simulink model "MPS_device_passive"  (R2018b)
settings: Solver=ode4  StartTime=0  StopTime=300  FixedStep=0.02  MaxStep=0.02  RelTol=1e-3  EnableMultiTasking=on
InitFcn:
  | %SSModel_calc
undefined symbols (not defined in the file): body, CentralPTOPreload, constraint, L, ML1Preload, ML2Preload, ML3Preload, ML4Preload, ML5Preload, ML6Preload, ML7Preload, ML8Preload, mrelative, pto, PTOrotation, SidePTO1Preload, SidePTO2Preload, SidePTO3Preload, SidePTO4Preload, simu, waves, X, Y, Z
libraries: nesl_utility x580, sm_lib x317, vrlib x72, WECSim_Lib x36
(part 2 of 27)

== system MPS_device_passive/ML4 ==
  Gimbal Fair4 : Subsystem  AncestorBlock=WECSim_Lib/Constraints/Rotational  mask(Constraints){constraint=constraint(1)}
      mask prompts: constraint "Constraint Name:"
      mask help:
      | Constraints the follower to rotational motion relative to the base, about
      | the constraint's Y-axis. Location is required and affects dynamics.
      |
      |
      | The variable name input below must be 'constraint(i)' where i=1,2,...
      | constraint(i) must be defined in the input file with the following fields:
      |
      |     .name (required)
      |             String.
      |             Constraint name. Must comply with Matlab's variable naming rules.
      |     .loc (required)
      |             3x1 vector [x y z] in meters.
      |             Constraint location. Default = [0 0 0]
      |     .orientation.z (optional)
      |             3x1 vector [x y z].
      |             Direction of the constraint's Z-coordinate. Default = [0 0 1]
      |     .orientation.y (optional)
      |             3x1 vector [x y z].
      |             Direction of the constraint's Y-coordinate. Default = [0 1 0]
      mask init: same as MPS_device_passive/Central tether/Gimbal F3
      settings: AttributesFormatString=%<constraint>
      mask Help:
      | Constraints the follower to rotational motion relative to the base, about
      | the constraint's Y-axis. Location is required and affects dynamics.
      | 
      | 
      | The variable name input below must be 'constraint(i)' where i=1,2,...
      | constraint(i) must be defined in the input file with the following fields:
      | 
      |     .name (required)
      |             String.
      |             Constraint name. Must comply with Matlab's variable naming rules.
      |     .loc (required)
      |             3x1 vector [x y z] in meters.
      |             Constraint location. Default = [0 0 0]
      |     .orientation.z (optional)
      |             3x1 vector [x y z].
      |             Direction of the constraint's Z-coordinate. Default = [0 0 1]
      |     .orientation.y (optional)
      |             3x1 vector [x y z].
      |             Direction of the constraint's Y-coordinate. Default = [0 1 0]
  ML4_preload : Constant  Value=ML4Preload
  Rigid Transform Anch4 : sm_lib/Frames and Transforms/Rigid Transform  TranslationMethod=None  TranslationStandardOffset=0  TranslationLengthUnit=m  TranslationStandardAxis=+Z  TranslationCartesianOffset=[0 0 0]  TranslationROffset=0  TranslationROffsetUnits=m  TranslationZOffset=0  TranslationZOffsetUnits=m  TranslationThetaOffset=0  TranslationThetaOffsetUnits=deg  RotationMethod=StandardAxis  RotationAngleUnits=rad  RotationStandardAxis=+Z  RotationAngle=pi-mrelative  RotationArbitraryAxis=[0 0 1]  FollAlignAxisA=+X  BaseAlignAxisA=+Y  FollAlignAxisB=+Y  BaseAlignAxisB=+Z  RotationSequenceAxes=FollowerAxes  RotationSequence=XYX  RotationSequenceAngles=[0 0 0]  RotationSequenceAnglesUnits=deg  RotationMatrix=[1 0 0; 0 1 0; 0 0 1]
  Rigid Transform F4P1 : sm_lib/Frames and Transforms/Rigid Transform  TranslationMethod=None  TranslationStandardOffset=0  TranslationLengthUnit=m  TranslationStandardAxis=+Z  TranslationCartesianOffset=[0 0 0]  TranslationROffset=0  TranslationROffsetUnits=m  TranslationZOffset=0  TranslationZOffsetUnits=m  TranslationThetaOffset=0  TranslationThetaOffsetUnits=deg  RotationMethod=StandardAxis  RotationAngleUnits=rad  RotationStandardAxis=+Z  RotationAngle=pi-mrelative  RotationArbitraryAxis=[0 0 1]  FollAlignAxisA=+X  BaseAlignAxisA=+Y  FollAlignAxisB=+Y  BaseAlignAxisB=+Z  RotationSequenceAxes=FollowerAxes  RotationSequence=XYX  RotationSequenceAngles=[0 0 0]  RotationSequenceAnglesUnits=deg  RotationMatrix=[1 0 0; 0 1 0; 0 0 1]
  Terminator3 : Terminator
  Translational PTO Actuation Force ML4 : Subsystem  AncestorBlock=WECSim_Lib/PTOs/Translational PTO Actuation Force  mask(PTO){pto=pto(9)}
      mask prompts: pto "PTO Name:"
      mask help:
      | Constraints the follower to translational motion relative to the base, in
      | the PTO's Z-direction and adds PTO stiffness and damping. Also applies a
      | user-defined force and outputs extension, velocity, and acceleration.
      |
      |
      | The variable name input below must be 'pto(i)' where i=1,2,...
      | pto(i) must be defined in the input file with the following fields:
      |
      |     .name (required)
      |             String.
      |             PTO name. Must comply with Matlab's variable naming rules.
      |     .loc (optional)
      |             3x1 vector [x y z] in meters.
      |             PTO location. Default = [0 0 0]
      |     .k (optional)
      |             Float.
      |             PTO linear spring stiffness. Default = 0
      |     .c (optional)
      |             Float.
      |             PTO linear damping coefficient. Default = 0
      |     .orientation.z (optional)
      |             3x1 vector [x y z].
      |             Direction of the PTO's Z-coordinate. Default = [0 0 1]
      |     .orientation.y (optional)
      |             3x1 vector [x y z].
      |             Direction of the PTO's Y-coordinate. Default = [0 1 0]
      mask init:
      | if exist('pto','var')
      |     h=[gcb '/output'];
      |     responseName=['pto' num2str(pto.ptoNum) '_out'];
      |     set_param(h,'VariableName',responseName);
      | end
      | 
      | pto.checkLoc('W');
      settings: AttributesFormatString=%<pto>
      mask Help:
      | Constraints the follower to translational motion relative to the base, in
      | the PTO's Z-direction and adds PTO stiffness and damping. Also applies a
      | user-defined force and outputs extension, velocity, and acceleration.
      | 
      | 
      | The variable name input below must be 'pto(i)' where i=1,2,...
      | pto(i) must be defined in the input file with the following fields:
      | 
      |     .name (required)
      |             String.
      |             PTO name. Must comply with Matlab's variable naming rules.
      |     .loc (optional)
      |             3x1 vector [x y z] in meters.
      |             PTO location. Default = [0 0 0]
      |     .k (optional)
      |             Float.
      |             PTO linear spring stiffness. Default = 0
      |     .c (optional)
      |             Float.
      |             PTO linear damping coefficient. Default = 0
      |     .orientation.z (optional)
      |             3x1 vector [x y z].
      |             Direction of the PTO's Z-coordinate. Default = [0 0 1]
      |     .orientation.y (optional)
      |             3x1 vector [x y z].
      |             Direction of the PTO's Y-coordinate. Default = [0 1 0]
  Universal Joint Anch4 : Subsystem  AncestorBlock=WECSim_Lib/Constraints/Rotational  mask(Constraints){constraint=constraint(18)}
      mask prompts: constraint "Constraint Name:"
      mask help:
      | Constraints the follower to rotational motion relative to the base, about
      | the constraint's Y-axis. Location is required and affects dynamics.
      |
      |
      | The variable name input below must be 'constraint(i)' where i=1,2,...
      | constraint(i) must be defined in the input file with the following fields:
      |
      |     .name (required)
      |             String.
      |             Constraint name. Must comply with Matlab's variable naming rules.
      |     .loc (required)
      |             3x1 vector [x y z] in meters.
      |             Constraint location. Default = [0 0 0]
      |     .orientation.z (optional)
      |             3x1 vector [x y z].
      |             Direction of the constraint's Z-coordinate. Default = [0 0 1]
      |     .orientation.y (optional)
      |             3x1 vector [x y z].
      |             Direction of the constraint's Y-coordinate. Default = [0 1 0]
      mask init: same as MPS_device_passive/Central tether/Gimbal F3
      settings: AttributesFormatString=%<constraint>
      mask Help:
      | Constraints the follower to rotational motion relative to the base, about
      | the constraint's Y-axis. Location is required and affects dynamics.
      | 
      | 
      | The variable name input below must be 'constraint(i)' where i=1,2,...
      | constraint(i) must be defined in the input file with the following fields:
      | 
      |     .name (required)
      |             String.
      |             Constraint name. Must comply with Matlab's variable naming rules.
      |     .loc (required)
      |             3x1 vector [x y z] in meters.
      |             Constraint location. Default = [0 0 0]
      |     .orientation.z (optional)
      |             3x1 vector [x y z].
      |             Direction of the constraint's Z-coordinate. Default = [0 0 1]
      |     .orientation.y (optional)
      |             3x1 vector [x y z].
      |             Direction of the constraint's Y-coordinate. Default = [0 1 0]
  VisuML1 : WECSim_Lib/Body Elements/Rigid Body  body=body(28)
      settings: AttributesFormatString=%<body>  SourceProductName=WEC-Sim
  VisuML2 : WECSim_Lib/Body Elements/Rigid Body  body=body(29)
      settings: AttributesFormatString=%<body>  SourceProductName=WEC-Sim
  VisuML4 : WECSim_Lib/Body Elements/Rigid Body  body=body(27)
      settings: AttributesFormatString=%<body>  SourceProductName=WEC-Sim
  Conn1 : PMIOPort  Side=Right
  Conn2 : PMIOPort  Port=2  Side=Left
  wires:
  ML4_preload/1 -> Translational PTO Actuation Force ML4/1(Force)
  Translational PTO Actuation Force ML4/1(Response) -> Terminator3/1
  connections:
  Gimbal Fair4/LConn1 -- Translational PTO Actuation Force ML4/RConn1 -- VisuML4/RConn1
  Rigid Transform F4P1/RConn1 -- Gimbal Fair4/RConn1
  Translational PTO Actuation Force ML4/LConn1 -- VisuML2/RConn1 -- Universal Joint Anch4/RConn1
  Universal Joint Anch4/LConn1 -- Rigid Transform Anch4/RConn1
  Rigid Transform F4P1/LConn1 -- VisuML1/RConn1 -- Conn2/RConn1
  Rigid Transform Anch4/LConn1 -- Conn1/RConn1

== system MPS_device_passive/ML5ver ==
  Gimbal Fair5 : Subsystem  AncestorBlock=WECSim_Lib/Constraints/Rotational  mask(Constraints){constraint=constraint(20)}
      mask prompts: constraint "Constraint Name:"
      mask help:
      | Constraints the follower to rotational motion relative to the base, about
      | the constraint's Y-axis. Location is required and affects dynamics.
      |
      |
      | The variable name input below must be 'constraint(i)' where i=1,2,...
      | constraint(i) must be defined in the input file with the following fields:
      |
      |     .name (required)
      |             String.
      |             Constraint name. Must comply with Matlab's variable naming rules.
      |     .loc (required)
      |             3x1 vector [x y z] in meters.
      |             Constraint location. Default = [0 0 0]
      |     .orientation.z (optional)
      |             3x1 vector [x y z].
      |             Direction of the constraint's Z-coordinate. Default = [0 0 1]
      |     .orientation.y (optional)
      |             3x1 vector [x y z].
      |             Direction of the constraint's Y-coordinate. Default = [0 1 0]
      mask init: same as MPS_device_passive/Central tether/Gimbal F3
      settings: AttributesFormatString=%<constraint>
      mask Help:
      | Constraints the follower to rotational motion relative to the base, about
      | the constraint's Y-axis. Location is required and affects dynamics.
      | 
      | 
      | The variable name input below must be 'constraint(i)' where i=1,2,...
      | constraint(i) must be defined in the input file with the following fields:
      | 
      |     .name (required)
      |             String.
      |             Constraint name. Must comply with Matlab's variable naming rules.
      |     .loc (required)
      |             3x1 vector [x y z] in meters.
      |             Constraint location. Default = [0 0 0]
      |     .orientation.z (optional)
      |             3x1 vector [x y z].
      |             Direction of the constraint's Z-coordinate. Default = [0 0 1]
      |     .orientation.y (optional)
      |             3x1 vector [x y z].
      |             Direction of the constraint's Y-coordinate. Default = [0 1 0]
  ML5_preload : Constant  Value=ML5Preload
  Rigid Transform Anch5 : sm_lib/Frames and Transforms/Rigid Transform  TranslationMethod=None  TranslationStandardOffset=0  TranslationLengthUnit=m  TranslationStandardAxis=+Z  TranslationCartesianOffset=[0 0 0]  TranslationROffset=0  TranslationROffsetUnits=m  TranslationZOffset=0  TranslationZOffsetUnits=m  TranslationThetaOffset=0  TranslationThetaOffsetUnits=deg  RotationMethod=StandardAxis  RotationAngleUnits=rad  RotationStandardAxis=+Z  RotationAngle=mrelative  RotationArbitraryAxis=[0 0 1]  FollAlignAxisA=+X  BaseAlignAxisA=+Y  FollAlignAxisB=+Y  BaseAlignAxisB=+Z  RotationSequenceAxes=FollowerAxes  RotationSequence=XYX  RotationSequenceAngles=[0 0 0]  RotationSequenceAnglesUnits=deg  RotationMatrix=[1 0 0; 0 1 0; 0 0 1]
  Rigid Transform Fair6 : sm_lib/Frames and Transforms/Rigid Transform  TranslationMethod=None  TranslationStandardOffset=0  TranslationLengthUnit=m  TranslationStandardAxis=+Z  TranslationCartesianOffset=[0 0 0]  TranslationROffset=0  TranslationROffsetUnits=m  TranslationZOffset=0  TranslationZOffsetUnits=m  TranslationThetaOffset=0  TranslationThetaOffsetUnits=deg  RotationMethod=StandardAxis  RotationAngleUnits=rad  RotationStandardAxis=+Z  RotationAngle=mrelative  RotationArbitraryAxis=[0 0 1]  FollAlignAxisA=+X  BaseAlignAxisA=+Y  FollAlignAxisB=+Y  BaseAlignAxisB=+Z  RotationSequenceAxes=FollowerAxes  RotationSequence=XYX  RotationSequenceAngles=[0 0 0]  RotationSequenceAnglesUnits=deg  RotationMatrix=[1 0 0; 0 1 0; 0 0 1]
  Terminator : Terminator
  Translational Actuation Force ML5 : Subsystem  AncestorBlock=WECSim_Lib/PTOs/Translational PTO Actuation Force  mask(PTO){pto=pto(10)}
      mask prompts: pto "PTO Name:"
      mask help:
      | Constraints the follower to translational motion relative to the base, in
      | the PTO's Z-direction and adds PTO stiffness and damping. Also applies a
      | user-defined force and outputs extension, velocity, and acceleration.
      |
      |
      | The variable name input below must be 'pto(i)' where i=1,2,...
      | pto(i) must be defined in the input file with the following fields:
      |
      |     .name (required)
      |             String.
      |             PTO name. Must comply with Matlab's variable naming rules.
      |     .loc (optional)
      |             3x1 vector [x y z] in meters.
      |             PTO location. Default = [0 0 0]
      |     .k (optional)
      |             Float.
      |             PTO linear spring stiffness. Default = 0
      |     .c (optional)
      |             Float.
      |             PTO linear damping coefficient. Default = 0
      |     .orientation.z (optional)
      |             3x1 vector [x y z].
      |             Direction of the PTO's Z-coordinate. Default = [0 0 1]
      |     .orientation.y (optional)
      |             3x1 vector [x y z].
      |             Direction of the PTO's Y-coordinate. Default = [0 1 0]
      mask init:
      | if exist('pto','var')
      |     h=[gcb '/output'];
      |     responseName=['pto' num2str(pto.ptoNum) '_out'];
      |     set_param(h,'VariableName',responseName);
      | end
      | 
      | pto.checkLoc('W');
      settings: AttributesFormatString=%<pto>
      mask Help:
      | Constraints the follower to translational motion relative to the base, in
      | the PTO's Z-direction and adds PTO stiffness and damping. Also applies a
      | user-defined force and outputs extension, velocity, and acceleration.
      | 
      | 
      | The variable name input below must be 'pto(i)' where i=1,2,...
      | pto(i) must be defined in the input file with the following fields:
      | 
      |     .name (required)
      |             String.
      |             PTO name. Must comply with Matlab's variable naming rules.
      |     .loc (optional)
      |             3x1 vector [x y z] in meters.
      |             PTO location. Default = [0 0 0]
      |     .k (optional)
      |             Float.
      |             PTO linear spring stiffness. Default = 0
      |     .c (optional)
      |             Float.
      |             PTO linear damping coefficient. Default = 0
      |     .orientation.z (optional)
      |             3x1 vector [x y z].
      |             Direction of the PTO's Z-coordinate. Default = [0 0 1]
      |     .orientation.y (optional)
      |             3x1 vector [x y z].
      |             Direction of the PTO's Y-coordinate. Default = [0 1 0]
  Universal Joint Anch5 : Subsystem  AncestorBlock=WECSim_Lib/Constraints/Rotational  mask(Constraints){constraint=constraint(19)}
      mask prompts: constraint "Constraint Name:"
      mask help:
      | Constraints the follower to rotational motion relative to the base, about
      | the constraint's Y-axis. Location is required and affects dynamics.
      |
      |
      | The variable name input below must be 'constraint(i)' where i=1,2,...
      | constraint(i) must be defined in the input file with the following fields:
      |
      |     .name (required)
      |             String.
      |             Constraint name. Must comply with Matlab's variable naming rules.
      |     .loc (required)
      |             3x1 vector [x y z] in meters.
      |             Constraint location. Default = [0 0 0]
      |     .orientation.z (optional)
      |             3x1 vector [x y z].
      |             Direction of the constraint's Z-coordinate. Default = [0 0 1]
      |     .orientation.y (optional)
      |             3x1 vector [x y z].
      |             Direction of the constraint's Y-coordinate. Default = [0 1 0]
      mask init: same as MPS_device_passive/Central tether/Gimbal F3
      settings: AttributesFormatString=%<constraint>
      mask Help:
      | Constraints the follower to rotational motion relative to the base, about
      | the constraint's Y-axis. Location is required and affects dynamics.
      | 
      | 
      | The variable name input below must be 'constraint(i)' where i=1,2,...
      | constraint(i) must be defined in the input file with the following fields:
      | 
      |     .name (required)
      |             String.
      |             Constraint name. Must comply with Matlab's variable naming rules.
      |     .loc (required)
      |             3x1 vector [x y z] in meters.
      |             Constraint location. Default = [0 0 0]
      |     .orientation.z (optional)
      |             3x1 vector [x y z].
      |             Direction of the constraint's Z-coordinate. Default = [0 0 1]
      |     .orientation.y (optional)
      |             3x1 vector [x y z].
      |             Direction of the constraint's Y-coordinate. Default = [0 1 0]
  VisuML5_1 : WECSim_Lib/Body Elements/Rigid Body  body=body(30)
      settings: AttributesFormatString=%<body>  SourceProductName=WEC-Sim
  VisuML5_2 : WECSim_Lib/Body Elements/Rigid Body  body=body(31)
      settings: AttributesFormatString=%<body>  SourceProductName=WEC-Sim
  VisuML5_3 : WECSim_Lib/Body Elements/Rigid Body  body=body(32)
      settings: AttributesFormatString=%<body>  SourceProductName=WEC-Sim
  Conn1 : PMIOPort  Side=Right
  Conn2 : PMIOPort  Port=2  Side=Left
  wires:
  Translational Actuation Force ML5/1(Response) -> Terminator/1
  ML5_preload/1 -> Translational Actuation Force ML5/1(Force)
  connections:
  VisuML5_1/RConn1 -- Translational Actuation Force ML5/RConn1 -- Gimbal Fair5/LConn1
  Translational Actuation Force ML5/LConn1 -- VisuML5_3/RConn1 -- Universal Joint Anch5/RConn1
  Universal Joint Anch5/LConn1 -- Rigid Transform Anch5/RConn1
  Rigid Transform Fair6/RConn1 -- Gimbal Fair5/RConn1
  Conn1/RConn1 -- Rigid Transform Anch5/LConn1
  Conn2/RConn1 -- VisuML5_2/RConn1 -- Rigid Transform Fair6/LConn1

== system MPS_device_passive/ML6ver ==
  Gimbal Fair6 : Subsystem  AncestorBlock=WECSim_Lib/Constraints/Rotational  mask(Constraints){constraint=constraint(22)}
      mask prompts: constraint "Constraint Name:"
      mask help:
      | Constraints the follower to rotational motion relative to the base, about
      | the constraint's Y-axis. Location is required and affects dynamics.
      |
      |
      | The variable name input below must be 'constraint(i)' where i=1,2,...
      | constraint(i) must be defined in the input file with the following fields:
      |
      |     .name (required)
      |             String.
      |             Constraint name. Must comply with Matlab's variable naming rules.
      |     .loc (required)
      |             3x1 vector [x y z] in meters.
      |             Constraint location. Default = [0 0 0]
      |     .orientation.z (optional)
      |             3x1 vector [x y z].
      |             Direction of the constraint's Z-coordinate. Default = [0 0 1]
      |     .orientation.y (optional)
      |             3x1 vector [x y z].
      |             Direction of the constraint's Y-coordinate. Default = [0 1 0]
      mask init: same as MPS_device_passive/Central tether/Gimbal F3
      settings: AttributesFormatString=%<constraint>
      mask Help:
      | Constraints the follower to rotational motion relative to the base, about
      | the constraint's Y-axis. Location is required and affects dynamics.
      | 
      | 
      | The variable name input below must be 'constraint(i)' where i=1,2,...
      | constraint(i) must be defined in the input file with the following fields:
      | 
      |     .name (required)
      |             String.
      |             Constraint name. Must comply with Matlab's variable naming rules.
      |     .loc (required)
      |             3x1 vector [x y z] in meters.
      |             Constraint location. Default = [0 0 0]
      |     .orientation.z (optional)
      |             3x1 vector [x y z].
      |             Direction of the constraint's Z-coordinate. Default = [0 0 1]
      |     .orientation.y (optional)
      |             3x1 vector [x y z].
      |             Direction of the constraint's Y-coordinate. Default = [0 1 0]
  ML6_preload : Constant  Value=ML6Preload
  Rigid Transform Anch6 : sm_lib/Frames and Transforms/Rigid Transform  TranslationMethod=None  TranslationStandardOffset=0  TranslationLengthUnit=m  TranslationStandardAxis=+Z  TranslationCartesianOffset=[0 0 0]  TranslationROffset=0  TranslationROffsetUnits=m  TranslationZOffset=0  TranslationZOffsetUnits=m  TranslationThetaOffset=0  TranslationThetaOffsetUnits=deg  RotationMethod=StandardAxis  RotationAngleUnits=rad  RotationStandardAxis=+Z  RotationAngle=-mrelative  RotationArbitraryAxis=[0 0 1]  FollAlignAxisA=+X  BaseAlignAxisA=+Y  FollAlignAxisB=+Y  BaseAlignAxisB=+Z  RotationSequenceAxes=FollowerAxes  RotationSequence=XYX  RotationSequenceAngles=[0 0 0]  RotationSequenceAnglesUnits=deg  RotationMatrix=[1 0 0; 0 1 0; 0 0 1]
  Rigid Transform Fair7 : sm_lib/Frames and Transforms/Rigid Transform  TranslationMethod=None  TranslationStandardOffset=0  TranslationLengthUnit=m  TranslationStandardAxis=+Z  TranslationCartesianOffset=[0 0 0]  TranslationROffset=0  TranslationROffsetUnits=m  TranslationZOffset=0  TranslationZOffsetUnits=m  TranslationThetaOffset=0  TranslationThetaOffsetUnits=deg  RotationMethod=StandardAxis  RotationAngleUnits=rad  RotationStandardAxis=+Z  RotationAngle=-mrelative  RotationArbitraryAxis=[0 0 1]  FollAlignAxisA=+X  BaseAlignAxisA=+Y  FollAlignAxisB=+Y  BaseAlignAxisB=+Z  RotationSequenceAxes=FollowerAxes  RotationSequence=XYX  RotationSequenceAngles=[0 0 0]  RotationSequenceAnglesUnits=deg  RotationMatrix=[1 0 0; 0 1 0; 0 0 1]
  Terminator1 : Terminator
  Translational PTO Actuation Force ML6 : Subsystem  AncestorBlock=WECSim_Lib/PTOs/Translational PTO Actuation Force  mask(PTO){pto=pto(11)}
      mask prompts: pto "PTO Name:"
      mask help:
      | Constraints the follower to translational motion relative to the base, in
      | the PTO's Z-direction and adds PTO stiffness and damping. Also applies a
      | user-defined force and outputs extension, velocity, and acceleration.
      |
      |
      | The variable name input below must be 'pto(i)' where i=1,2,...
      | pto(i) must be defined in the input file with the following fields:
      |
      |     .name (required)
      |             String.
      |             PTO name. Must comply with Matlab's variable naming rules.
      |     .loc (optional)
      |             3x1 vector [x y z] in meters.
      |             PTO location. Default = [0 0 0]
      |     .k (optional)
      |             Float.
      |             PTO linear spring stiffness. Default = 0
      |     .c (optional)
      |             Float.
      |             PTO linear damping coefficient. Default = 0
      |     .orientation.z (optional)
      |             3x1 vector [x y z].
      |             Direction of the PTO's Z-coordinate. Default = [0 0 1]
      |     .orientation.y (optional)
      |             3x1 vector [x y z].
      |             Direction of the PTO's Y-coordinate. Default = [0 1 0]
      mask init:
      | if exist('pto','var')
      |     h=[gcb '/output'];
      |     responseName=['pto' num2str(pto.ptoNum) '_out'];
      |     set_param(h,'VariableName',responseName);
      | end
      | 
      | pto.checkLoc('W');
      settings: AttributesFormatString=%<pto>
      mask Help:
      | Constraints the follower to translational motion relative to the base, in
      | the PTO's Z-direction and adds PTO stiffness and damping. Also applies a
      | user-defined force and outputs extension, velocity, and acceleration.
      | 
      | 
      | The variable name input below must be 'pto(i)' where i=1,2,...
      | pto(i) must be defined in the input file with the following fields:
      | 
      |     .name (required)
      |             String.
      |             PTO name. Must comply with Matlab's variable naming rules.
      |     .loc (optional)
      |             3x1 vector [x y z] in meters.
      |             PTO location. Default = [0 0 0]
      |     .k (optional)
      |             Float.
      |             PTO linear spring stiffness. Default = 0
      |     .c (optional)
      |             Float.
      |             PTO linear damping coefficient. Default = 0
      |     .orientation.z (optional)
      |             3x1 vector [x y z].
      |             Direction of the PTO's Z-coordinate. Default = [0 0 1]
      |     .orientation.y (optional)
      |             3x1 vector [x y z].
      |             Direction of the PTO's Y-coordinate. Default = [0 1 0]
  Universal Joint Anch6 : Subsystem  AncestorBlock=WECSim_Lib/Constraints/Rotational  mask(Constraints){constraint=constraint(21)}
      mask prompts: constraint "Constraint Name:"
      mask help:
      | Constraints the follower to rotational motion relative to the base, about
      | the constraint's Y-axis. Location is required and affects dynamics.
      |
      |
      | The variable name input below must be 'constraint(i)' where i=1,2,...
      | constraint(i) must be defined in the input file with the following fields:
      |
      |     .name (required)
      |             String.
      |             Constraint name. Must comply with Matlab's variable naming rules.
      |     .loc (required)
      |             3x1 vector [x y z] in meters.
      |             Constraint location. Default = [0 0 0]
      |     .orientation.z (optional)
      |             3x1 vector [x y z].
      |             Direction of the constraint's Z-coordinate. Default = [0 0 1]
      |     .orientation.y (optional)
      |             3x1 vector [x y z].
      |             Direction of the constraint's Y-coordinate. Default = [0 1 0]
      mask init: same as MPS_device_passive/Central tether/Gimbal F3
      settings: AttributesFormatString=%<constraint>
      mask Help:
      | Constraints the follower to rotational motion relative to the base, about
      | the constraint's Y-axis. Location is required and affects dynamics.
      | 
      | 
      | The variable name input below must be 'constraint(i)' where i=1,2,...
      | constraint(i) must be defined in the input file with the following fields:
      | 
      |     .name (required)
      |             String.
      |             Constraint name. Must comply with Matlab's variable naming rules.
      |     .loc (required)
      |             3x1 vector [x y z] in meters.
      |             Constraint location. Default = [0 0 0]
      |     .orientation.z (optional)
      |             3x1 vector [x y z].
      |             Direction of the constraint's Z-coordinate. Default = [0 0 1]
      |     .orientation.y (optional)
      |             3x1 vector [x y z].
      |             Direction of the constraint's Y-coordinate. Default = [0 1 0]
  VisuML6_1 : WECSim_Lib/Body Elements/Rigid Body  body=body(33)
      settings: AttributesFormatString=%<body>  SourceProductName=WEC-Sim
  VisuML6_2 : WECSim_Lib/Body Elements/Rigid Body  body=body(34)
      settings: AttributesFormatString=%<body>  SourceProductName=WEC-Sim
  VisuML6_3 : WECSim_Lib/Body Elements/Rigid Body  body=body(35)
      settings: AttributesFormatString=%<body>  SourceProductName=WEC-Sim
  Conn1 : PMIOPort  Side=Right
  Conn2 : PMIOPort  Port=2  Side=Left
  wires:
  ML6_preload/1 -> Translational PTO Actuation Force ML6/1(Force)
  Translational PTO Actuation Force ML6/1(Response) -> Terminator1/1
  connections:
  VisuML6_1/RConn1 -- Translational PTO Actuation Force ML6/RConn1 -- Gimbal Fair6/LConn1
  Rigid Transform Fair7/RConn1 -- Gimbal Fair6/RConn1
  Translational PTO Actuation Force ML6/LConn1 -- VisuML6_3/RConn1 -- Universal Joint Anch6/RConn1
  Universal Joint Anch6/LConn1 -- Rigid Transform Anch6/RConn1
  Conn1/RConn1 -- Rigid Transform Anch6/LConn1
  Conn2/RConn1 -- Rigid Transform Fair7/LConn1 -- VisuML6_2/RConn1

== system MPS_device_passive/ML7ver ==
  Gimbal Fair7 : Subsystem  AncestorBlock=WECSim_Lib/Constraints/Rotational  mask(Constraints){constraint=constraint(24)}
      mask prompts: constraint "Constraint Name:"
      mask help:
      | Constraints the follower to rotational motion relative to the base, about
      | the constraint's Y-axis. Location is required and affects dynamics.
      |
      |
      | The variable name input below must be 'constraint(i)' where i=1,2,...
      | constraint(i) must be defined in the input file with the following fields:
      |
      |     .name (required)
      |             String.
      |             Constraint name. Must comply with Matlab's variable naming rules.
      |     .loc (required)
      |             3x1 vector [x y z] in meters.
      |             Constraint location. Default = [0 0 0]
      |     .orientation.z (optional)
      |             3x1 vector [x y z].
      |             Direction of the constraint's Z-coordinate. Default = [0 0 1]
      |     .orientation.y (optional)
      |             3x1 vector [x y z].
      |             Direction of the constraint's Y-coordinate. Default = [0 1 0]
      mask init: same as MPS_device_passive/Central tether/Gimbal F3
      settings: AttributesFormatString=%<constraint>
      mask Help:
      | Constraints the follower to rotational motion relative to the base, about
      | the constraint's Y-axis. Location is required and affects dynamics.
      | 
      | 
      | The variable name input below must be 'constraint(i)' where i=1,2,...
      | constraint(i) must be defined in the input file with the following fields:
      | 
      |     .name (required)
      |             String.
      |             Constraint name. Must comply with Matlab's variable naming rules.
      |     .loc (required)
      |             3x1 vector [x y z] in meters.
      |             Constraint location. Default = [0 0 0]
      |     .orientation.z (optional)
      |             3x1 vector [x y z].
      |             Direction of the constraint's Z-coordinate. Default = [0 0 1]
      |     .orientation.y (optional)
      |             3x1 vector [x y z].
      |             Direction of the constraint's Y-coordinate. Default = [0 1 0]
  ML7_preload : Constant  Value=ML7Preload
  Rigid Transform Anch7 : sm_lib/Frames and Transforms/Rigid Transform  TranslationMethod=None  TranslationStandardOffset=0  TranslationLengthUnit=m  TranslationStandardAxis=+Z  TranslationCartesianOffset=[0 0 0]  TranslationROffset=0  TranslationROffsetUnits=m  TranslationZOffset=0  TranslationZOffsetUnits=m  TranslationThetaOffset=0  TranslationThetaOffsetUnits=deg  RotationMethod=StandardAxis  RotationAngleUnits=rad  RotationStandardAxis=+Z  RotationAngle=-pi+mrelative  RotationArbitraryAxis=[0 0 1]  FollAlignAxisA=+X  BaseAlignAxisA=+Y  FollAlignAxisB=+Y  BaseAlignAxisB=+Z  RotationSequenceAxes=FollowerAxes  RotationSequence=XYX  RotationSequenceAngles=[0 0 0]  RotationSequenceAnglesUnits=deg  RotationMatrix=[1 0 0; 0 1 0; 0 0 1]
  Rigid Transform Fair8 : sm_lib/Frames and Transforms/Rigid Transform  TranslationMethod=None  TranslationStandardOffset=0  TranslationLengthUnit=m  TranslationStandardAxis=+Z  TranslationCartesianOffset=[0 0 0]  TranslationROffset=0  TranslationROffsetUnits=m  TranslationZOffset=0  TranslationZOffsetUnits=m  TranslationThetaOffset=0  TranslationThetaOffsetUnits=deg  RotationMethod=StandardAxis  RotationAngleUnits=rad  RotationStandardAxis=+Z  RotationAngle=-pi+mrelative  RotationArbitraryAxis=[0 0 1]  FollAlignAxisA=+X  BaseAlignAxisA=+Y  FollAlignAxisB=+Y  BaseAlignAxisB=+Z  RotationSequenceAxes=FollowerAxes  RotationSequence=XYX  RotationSequenceAngles=[0 0 0]  RotationSequenceAnglesUnits=deg  RotationMatrix=[1 0 0; 0 1 0; 0 0 1]
  Terminator2 : Terminator
  Translational PTO Actuation Force ML7 : Subsystem  AncestorBlock=WECSim_Lib/PTOs/Translational PTO Actuation Force  mask(PTO){pto=pto(12)}
      mask prompts: pto "PTO Name:"
      mask help:
      | Constraints the follower to translational motion relative to the base, in
      | the PTO's Z-direction and adds PTO stiffness and damping. Also applies a
      | user-defined force and outputs extension, velocity, and acceleration.
      |
      |
      | The variable name input below must be 'pto(i)' where i=1,2,...
      | pto(i) must be defined in the input file with the following fields:
      |
      |     .name (required)
      |             String.
      |             PTO name. Must comply with Matlab's variable naming rules.
      |     .loc (optional)
      |             3x1 vector [x y z] in meters.
      |             PTO location. Default = [0 0 0]
      |     .k (optional)
      |             Float.
      |             PTO linear spring stiffness. Default = 0
      |     .c (optional)
      |             Float.
      |             PTO linear damping coefficient. Default = 0
      |     .orientation.z (optional)
      |             3x1 vector [x y z].
      |             Direction of the PTO's Z-coordinate. Default = [0 0 1]
      |     .orientation.y (optional)
      |             3x1 vector [x y z].
      |             Direction of the PTO's Y-coordinate. Default = [0 1 0]
      mask init:
      | if exist('pto','var')
      |     h=[gcb '/output'];
      |     responseName=['pto' num2str(pto.ptoNum) '_out'];
      |     set_param(h,'VariableName',responseName);
      | end
      | 
      | pto.checkLoc('W');
      settings: AttributesFormatString=%<pto>
      mask Help:
      | Constraints the follower to translational motion relative to the base, in
      | the PTO's Z-direction and adds PTO stiffness and damping. Also applies a
      | user-defined force and outputs extension, velocity, and acceleration.
      | 
      | 
      | The variable name input below must be 'pto(i)' where i=1,2,...
      | pto(i) must be defined in the input file with the following fields:
      | 
      |     .name (required)
      |             String.
      |             PTO name. Must comply with Matlab's variable naming rules.
      |     .loc (optional)
      |             3x1 vector [x y z] in meters.
      |             PTO location. Default = [0 0 0]
      |     .k (optional)
      |             Float.
      |             PTO linear spring stiffness. Default = 0
      |     .c (optional)
      |             Float.
      |             PTO linear damping coefficient. Default = 0
      |     .orientation.z (optional)
      |             3x1 vector [x y z].
      |             Direction of the PTO's Z-coordinate. Default = [0 0 1]
      |     .orientation.y (optional)
      |             3x1 vector [x y z].
      |             Direction of the PTO's Y-coordinate. Default = [0 1 0]
  Universal Joint Anch7 : Subsystem  AncestorBlock=WECSim_Lib/Constraints/Rotational  mask(Constraints){constraint=constraint(23)}
      mask prompts: constraint "Constraint Name:"
      mask help:
      | Constraints the follower to rotational motion relative to the base, about
      | the constraint's Y-axis. Location is required and affects dynamics.
      |
      |
      | The variable name input below must be 'constraint(i)' where i=1,2,...
      | constraint(i) must be defined in the input file with the following fields:
      |
      |     .name (required)
      |             String.
      |             Constraint name. Must comply with Matlab's variable naming rules.
      |     .loc (required)
      |             3x1 vector [x y z] in meters.
      |             Constraint location. Default = [0 0 0]
      |     .orientation.z (optional)
      |             3x1 vector [x y z].
      |             Direction of the constraint's Z-coordinate. Default = [0 0 1]
      |     .orientation.y (optional)
      |             3x1 vector [x y z].
      |             Direction of the constraint's Y-coordinate. Default = [0 1 0]
      mask init: same as MPS_device_passive/Central tether/Gimbal F3
      settings: AttributesFormatString=%<constraint>
      mask Help:
      | Constraints the follower to rotational motion relative to the base, about
      | the constraint's Y-axis. Location is required and affects dynamics.
      | 
      | 
      | The variable name input below must be 'constraint(i)' where i=1,2,...
      | constraint(i) must be defined in the input file with the following fields:
      | 
      |     .name (required)
      |             String.
      |             Constraint name. Must comply with Matlab's variable naming rules.
      |     .loc (required)
      |             3x1 vector [x y z] in meters.
      |             Constraint location. Default = [0 0 0]
      |     .orientation.z (optional)
      |             3x1 vector [x y z].
      |             Direction of the constraint's Z-coordinate. Default = [0 0 1]
      |     .orientation.y (optional)
      |             3x1 vector [x y z].
      |             Direction of the constraint's Y-coordinate. Default = [0 1 0]
  VisuML7_1 : WECSim_Lib/Body Elements/Rigid Body  body=body(36)
      settings: AttributesFormatString=%<body>  SourceProductName=WEC-Sim
  VisuML7_2 : WECSim_Lib/Body Elements/Rigid Body  body=body(37)
      settings: AttributesFormatString=%<body>  SourceProductName=WEC-Sim
  VisuML7_3 : WECSim_Lib/Body Elements/Rigid Body  body=body(38)
      settings: AttributesFormatString=%<body>  SourceProductName=WEC-Sim
  Conn1 : PMIOPort  Side=Right
  Conn2 : PMIOPort  Port=2  Side=Left
  wires:
  Translational PTO Actuation Force ML7/1(Response) -> Terminator2/1
  ML7_preload/1 -> Translational PTO Actuation Force ML7/1(Force1)
  connections:
  Gimbal Fair7/LConn1 -- Translational PTO Actuation Force ML7/RConn1 -- VisuML7_1/RConn1
  Rigid Transform Fair8/RConn1 -- Gimbal Fair7/RConn1
  Translational PTO Actuation Force ML7/LConn1 -- VisuML7_3/RConn1 -- Universal Joint Anch7/RConn1
  Universal Joint Anch7/LConn1 -- Rigid Transform Anch7/RConn1
  Conn1/RConn1 -- Rigid Transform Anch7/LConn1
  Conn2/RConn1 -- VisuML7_2/RConn1 -- Rigid Transform Fair8/LConn1

== system MPS_device_passive/ML8ver ==
  Gimbal Fair9 : Subsystem  AncestorBlock=WECSim_Lib/Constraints/Rotational  mask(Constraints){constraint=constraint(26)}
      mask prompts: constraint "Constraint Name:"
      mask help:
      | Constraints the follower to rotational motion relative to the base, about
      | the constraint's Y-axis. Location is required and affects dynamics.
      |
      |
      | The variable name input below must be 'constraint(i)' where i=1,2,...
      | constraint(i) must be defined in the input file with the following fields:
      |
      |     .name (required)
      |             String.
      |             Constraint name. Must comply with Matlab's variable naming rules.
      |     .loc (required)
      |             3x1 vector [x y z] in meters.
      |             Constraint location. Default = [0 0 0]
      |     .orientation.z (optional)
      |             3x1 vector [x y z].
      |             Direction of the constraint's Z-coordinate. Default = [0 0 1]
      |     .orientation.y (optional)
      |             3x1 vector [x y z].
      |             Direction of the constraint's Y-coordinate. Default = [0 1 0]
      mask init: same as MPS_device_passive/Central tether/Gimbal F3
      settings: AttributesFormatString=%<constraint>
      mask Help:
      | Constraints the follower to rotational motion relative to the base, about
      | the constraint's Y-axis. Location is required and affects dynamics.
      | 
      | 
      | The variable name input below must be 'constraint(i)' where i=1,2,...
      | constraint(i) must be defined in the input file with the following fields:
      | 
      |     .name (required)
      |             String.
      |             Constraint name. Must comply with Matlab's variable naming rules.
      |     .loc (required)
      |             3x1 vector [x y z] in meters.
      |             Constraint location. Default = [0 0 0]
      |     .orientation.z (optional)
      |             3x1 vector [x y z].
      |             Direction of the constraint's Z-coordinate. Default = [0 0 1]
      |     .orientation.y (optional)
      |             3x1 vector [x y z].
      |             Direction of the constraint's Y-coordinate. Default = [0 1 0]
  ML8_preload : Constant  Value=ML8Preload
  Rigid Transform Anch9 : sm_lib/Frames and Transforms/Rigid Transform  TranslationMethod=None  TranslationStandardOffset=0  TranslationLengthUnit=m  TranslationStandardAxis=+Z  TranslationCartesianOffset=[0 0 0]  TranslationROffset=0  TranslationROffsetUnits=m  TranslationZOffset=0  TranslationZOffsetUnits=m  TranslationThetaOffset=0  TranslationThetaOffsetUnits=deg  RotationMethod=StandardAxis  RotationAngleUnits=rad  RotationStandardAxis=+Z  RotationAngle=pi-mrelative  RotationArbitraryAxis=[0 0 1]  FollAlignAxisA=+X  BaseAlignAxisA=+Y  FollAlignAxisB=+Y  BaseAlignAxisB=+Z  RotationSequenceAxes=FollowerAxes  RotationSequence=XYX  RotationSequenceAngles=[0 0 0]  RotationSequenceAnglesUnits=deg  RotationMatrix=[1 0 0; 0 1 0; 0 0 1]
  Rigid Transform F4P9 : sm_lib/Frames and Transforms/Rigid Transform  TranslationMethod=None  TranslationStandardOffset=0  TranslationLengthUnit=m  TranslationStandardAxis=+Z  TranslationCartesianOffset=[0 0 0]  TranslationROffset=0  TranslationROffsetUnits=m  TranslationZOffset=0  TranslationZOffsetUnits=m  TranslationThetaOffset=0  TranslationThetaOffsetUnits=deg  RotationMethod=StandardAxis  RotationAngleUnits=rad  RotationStandardAxis=+Z  RotationAngle=pi-mrelative  RotationArbitraryAxis=[0 0 1]  FollAlignAxisA=+X  BaseAlignAxisA=+Y  FollAlignAxisB=+Y  BaseAlignAxisB=+Z  RotationSequenceAxes=FollowerAxes  RotationSequence=XYX  RotationSequenceAngles=[0 0 0]  RotationSequenceAnglesUnits=deg  RotationMatrix=[1 0 0; 0 1 0; 0 0 1]
  Terminator3 : Terminator
  Translational PTO Actuation Force ML9 : Subsystem  AncestorBlock=WECSim_Lib/PTOs/Translational PTO Actuation Force  mask(PTO){pto=pto(13)}
      mask prompts: pto "PTO Name:"
      mask help:
      | Constraints the follower to translational motion relative to the base, in
      | the PTO's Z-direction and adds PTO stiffness and damping. Also applies a
      | user-defined force and outputs extension, velocity, and acceleration.
      |
      |
      | The variable name input below must be 'pto(i)' where i=1,2,...
      | pto(i) must be defined in the input file with the following fields:
      |
      |     .name (required)
      |             String.
      |             PTO name. Must comply with Matlab's variable naming rules.
      |     .loc (optional)
      |             3x1 vector [x y z] in meters.
      |             PTO location. Default = [0 0 0]
      |     .k (optional)
      |             Float.
      |             PTO linear spring stiffness. Default = 0
      |     .c (optional)
      |             Float.
      |             PTO linear damping coefficient. Default = 0
      |     .orientation.z (optional)
      |             3x1 vector [x y z].
      |             Direction of the PTO's Z-coordinate. Default = [0 0 1]
      |     .orientation.y (optional)
      |             3x1 vector [x y z].
      |             Direction of the PTO's Y-coordinate. Default = [0 1 0]
      mask init:
      | if exist('pto','var')
      |     h=[gcb '/output'];
      |     responseName=['pto' num2str(pto.ptoNum) '_out'];
      |     set_param(h,'VariableName',responseName);
      | end
      | 
      | pto.checkLoc('W');
      settings: AttributesFormatString=%<pto>
      mask Help:
      | Constraints the follower to translational motion relative to the base, in
      | the PTO's Z-direction and adds PTO stiffness and damping. Also applies a
      | user-defined force and outputs extension, velocity, and acceleration.
      | 
      | 
      | The variable name input below must be 'pto(i)' where i=1,2,...
      | pto(i) must be defined in the input file with the following fields:
      | 
      |     .name (required)
      |             String.
      |             PTO name. Must comply with Matlab's variable naming rules.
      |     .loc (optional)
      |             3x1 vector [x y z] in meters.
      |             PTO location. Default = [0 0 0]
      |     .k (optional)
      |             Float.
      |             PTO linear spring stiffness. Default = 0
      |     .c (optional)
      |             Float.
      |             PTO linear damping coefficient. Default = 0
      |     .orientation.z (optional)
      |             3x1 vector [x y z].
      |             Direction of the PTO's Z-coordinate. Default = [0 0 1]
      |     .orientation.y (optional)
      |             3x1 vector [x y z].
      |             Direction of the PTO's Y-coordinate. Default = [0 1 0]
  Universal Joint Anch9 : Subsystem  AncestorBlock=WECSim_Lib/Constraints/Rotational  mask(Constraints){constraint=constraint(25)}
      mask prompts: constraint "Constraint Name:"
      mask help:
      | Constraints the follower to rotational motion relative to the base, about
      | the constraint's Y-axis. Location is required and affects dynamics.
      |
      |
      | The variable name input below must be 'constraint(i)' where i=1,2,...
      | constraint(i) must be defined in the input file with the following fields:
      |
      |     .name (required)
      |             String.
      |             Constraint name. Must comply with Matlab's variable naming rules.
      |     .loc (required)
      |             3x1 vector [x y z] in meters.
      |             Constraint location. Default = [0 0 0]
      |     .orientation.z (optional)
      |             3x1 vector [x y z].
      |             Direction of the constraint's Z-coordinate. Default = [0 0 1]
      |     .orientation.y (optional)
      |             3x1 vector [x y z].
      |             Direction of the constraint's Y-coordinate. Default = [0 1 0]
      mask init: same as MPS_device_passive/Central tether/Gimbal F3
      settings: AttributesFormatString=%<constraint>
      mask Help:
      | Constraints the follower to rotational motion relative to the base, about
      | the constraint's Y-axis. Location is required and affects dynamics.
      | 
      | 
      | The variable name input below must be 'constraint(i)' where i=1,2,...
      | constraint(i) must be defined in the input file with the following fields:
      | 
      |     .name (required)
      |             String.
      |             Constraint name. Must comply with Matlab's variable naming rules.
      |     .loc (required)
      |             3x1 vector [x y z] in meters.
      |             Constraint location. Default = [0 0 0]
      |     .orientation.z (optional)
      |             3x1 vector [x y z].
      |             Direction of the constraint's Z-coordinate. Default = [0 0 1]
      |     .orientation.y (optional)
      |             3x1 vector [x y z].
      |             Direction of the constraint's Y-coordinate. Default = [0 1 0]
  VisuML9_1 : WECSim_Lib/Body Elements/Rigid Body  body=body(39)
      settings: AttributesFormatString=%<body>  SourceProductName=WEC-Sim
  VisuML9_2 : WECSim_Lib/Body Elements/Rigid Body  body=body(40)
      settings: AttributesFormatString=%<body>  SourceProductName=WEC-Sim
  VisuML9_3 : WECSim_Lib/Body Elements/Rigid Body  body=body(41)
      settings: AttributesFormatString=%<body>  SourceProductName=WEC-Sim
  Conn1 : PMIOPort  Side=Right
  Conn2 : PMIOPort  Port=2  Side=Left
  wires:
  ML8_preload/1 -> Translational PTO Actuation Force ML9/1(Force)
  Translational PTO Actuation Force ML9/1(Response) -> Terminator3/1
  connections:
  Gimbal Fair9/LConn1 -- Translational PTO Actuation Force ML9/RConn1 -- VisuML9_1/RConn1
  Rigid Transform F4P9/RConn1 -- Gimbal Fair9/RConn1
  Translational PTO Actuation Force ML9/LConn1 -- VisuML9_3/RConn1 -- Universal Joint Anch9/RConn1
  Universal Joint Anch9/LConn1 -- Rigid Transform Anch9/RConn1
  Rigid Transform F4P9/LConn1 -- VisuML9_2/RConn1 -- Conn2/RConn1
  Rigid Transform Anch9/LConn1 -- Conn1/RConn1
